simulink model "scdairframe"  (Simulink 6.0)
settings: Solver=ode45  SolverMode=SingleTasking  StartTime=0.0  StopTime=10.0  RelTol=1e-3  AbsTol=1e-6
PreLoadFcn:
  | aero_guid_dat
undefined symbols (not defined in the file or in its folder): Cm_alpha, Cm_el, Cm_q, Cx_alpha, Cz_alpha, Cz_el, d_ref, g, h_ini, S_ref, Thrust, x_ini
libraries: aerospace x3
settings Model: Creator=The Mathworks Inc.  LastModifiedBy=jglass  ExtModeTrigMode=oneshot  ExtModeArmWhenConnect=off  ExtModeAutoUpdateStatusClock=off
settings DataIOCC: LimitDataPoints=off  SignalLoggingName=sigsOut
settings OptimizationCC: BlockReduction=off  BooleanDataType=off
settings DebuggingCC: CheckExecutionContextPreStartOutputMsg=on  CheckExecutionContextRuntimeOutputMsg=on  SolverPrmCheckMsg=none
settings HardwareCC: TargetUnknown=on
settings SFSimCC: SFSimApplyToAllLibs=on  SFSimBuildMode=Incremental

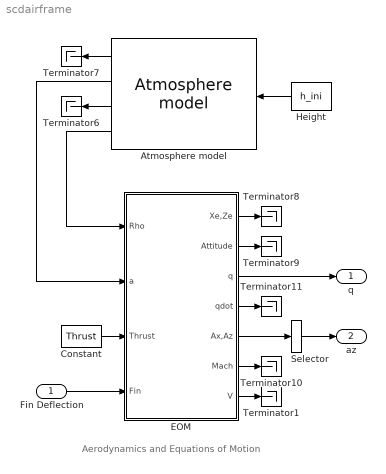
== system scdairframe ==
  note: Aerodynamics and Equations of Motion
  Fin Deflection : Inport  LatchInput=off
  Atmosphere model : aerospace/Atmosphere/Atmosphere model  Orientation=left
  Constant : Constant  Value=Thrust
  EOM : Subsystem  PropExecContextAcrossSSBoundary=on
  Height : Constant  Orientation=left  Value=h_ini
  Selector : Selector  Elements=[2]  InputPortWidth=2
  Terminator{1,6..11} (7 alike) : Terminator
  q : Outport  InitialOutput=0
  az : Outport  Port=2  InitialOutput=0
  wires:
  Height/1 -> Atmosphere model/1
  Atmosphere model/1 -> Terminator7/1
  Atmosphere model/3 -> Terminator6/1
  Constant/1 -> EOM/3(Thrust)
  Fin Deflection/1 -> EOM/4(Fin)
  EOM/1(Xe,Ze) -> Terminator8/1
  EOM/2(Attitude) -> Terminator9/1
  EOM/3(q) -> q/1
  EOM/4(qdot) -> Terminator11/1
  EOM/5(Ax,Az) -> Selector/1
  EOM/6(Mach) -> Terminator10/1
  Atmosphere model/4 -> EOM/1(Rho)
  Atmosphere model/2 -> EOM/2(a)
  Selector/1 -> az/1
  EOM/7(V) -> Terminator1/1

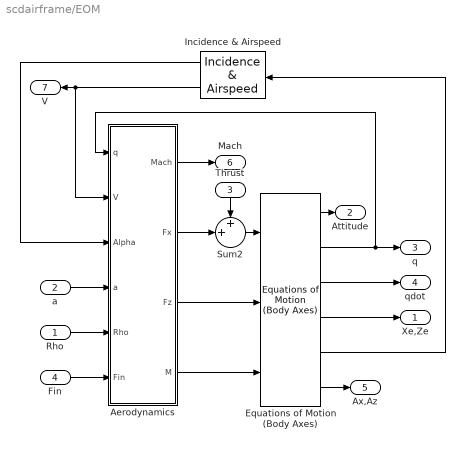
== system scdairframe/EOM ==
  Rho : Inport  LatchInput=off
  a : Inport  Port=2  LatchInput=off
  Thrust : Inport  Orientation=down  Port=3  LatchInput=off
  Fin : Inport  Port=4  LatchInput=off
  " Equations of Motion (Body Axes)" : aerospace/3DoF Equations of Motion / Equations of Motion (Body Axes)  v_ini=v_ini  theta_ini=theta_ini  alpha_ini=alpha_ini  q_ini=q_ini  pos_ini=[x_ini -h_ini]  mass=mass  Iyy=Iyy  g=g
  Aerodynamics : Subsystem  PropExecContextAcrossSSBoundary=on
  Incidence & Airspeed : aerospace/3DoF Equations of Motion /Incidence  & Airspeed  Orientation=left
  Sum2 : Sum  Inputs=++|  SaturateOnIntegerOverflow=on  InputSameDT=on
  Xe,Ze : Outport  InitialOutput=0
  Attitude : Outport  Port=2  InitialOutput=0
  q : Outport  Port=3  InitialOutput=0
  qdot : Outport  Port=4  InitialOutput=0
  Ax,Az : Outport  Port=5  InitialOutput=0
  Mach : Outport  Port=6  InitialOutput=0
  V : Outport  Orientation=left  Port=7  InitialOutput=0
  wires:
  " Equations of Motion (Body Axes)"/5 -> Incidence & Airspeed/1
  " Equations of Motion (Body Axes)"/6 -> Ax,Az/1
  " Equations of Motion (Body Axes)"/4 -> Xe,Ze/1
  " Equations of Motion (Body Axes)"/1 -> Attitude/1
  " Equations of Motion (Body Axes)"/3 -> qdot/1
  " Equations of Motion (Body Axes)"/2 -> Aerodynamics/1(q), q/1
  Thrust/1 -> Sum2/1
  Aerodynamics/2(Fx) -> Sum2/2
  Aerodynamics/3(Fz) -> " Equations of Motion (Body Axes)"/2
  Incidence & Airspeed/2 -> Aerodynamics/2(V), V/1
  Fin/1 -> Aerodynamics/6(Fin)
  a/1 -> Aerodynamics/4(a)
  Rho/1 -> Aerodynamics/5(Rho)
  Incidence & Airspeed/1 -> Aerodynamics/3(Alpha)
  Sum2/1 -> " Equations of Motion (Body Axes)"/1
  Aerodynamics/4(" M") -> " Equations of Motion (Body Axes)"/3
  Aerodynamics/1(" Mach") -> Mach/1

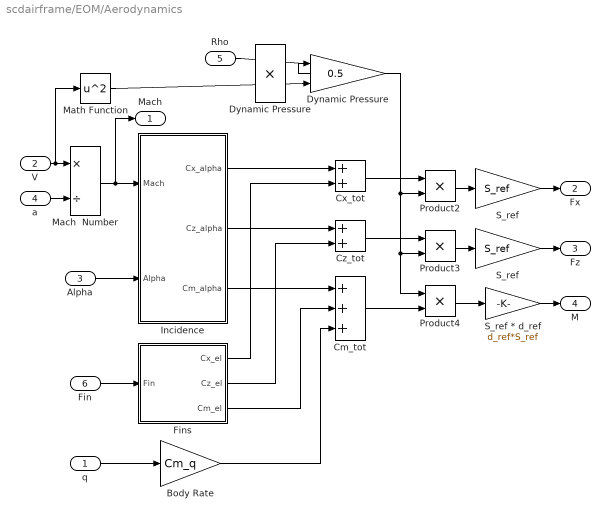
== system scdairframe/EOM/Aerodynamics ==
  q : Inport  LatchInput=off
  V : Inport  Port=2  LatchInput=off
  Alpha : Inport  Port=3  LatchInput=off
  a : Inport  Port=4  LatchInput=off
  Rho : Inport  Port=5  LatchInput=off
  Fin : Inport  Port=6  LatchInput=off
  Body Rate : Gain  Gain=Cm_q  SaturateOnIntegerOverflow=on
  Cm_tot : Sum  Inputs=+++  SaturateOnIntegerOverflow=on  InputSameDT=on
  Cx_tot : Sum  SaturateOnIntegerOverflow=on  InputSameDT=on
  Cz_tot : Sum  SaturateOnIntegerOverflow=on  InputSameDT=on
  Dynamic Pressure : Gain  Gain=0.5  SaturateOnIntegerOverflow=on
  Dynamic Pressure : Product  SaturateOnIntegerOverflow=on  InputSameDT=on
  Fins : Subsystem  PropExecContextAcrossSSBoundary=on
  Incidence : Subsystem  PropExecContextAcrossSSBoundary=on
  Mach  Number : Product  Inputs=*/  SaturateOnIntegerOverflow=on  InputSameDT=on
  Math Function : Math  Operator=square  SaturateOnIntegerOverflow=on
  Product2 : Product  SaturateOnIntegerOverflow=on  InputSameDT=on
  Product3 : Product  SaturateOnIntegerOverflow=on  InputSameDT=on
  Product4 : Product  SaturateOnIntegerOverflow=on  InputSameDT=on
  S_ref : Gain  Gain=S_ref  SaturateOnIntegerOverflow=on
  S_ref * d_ref : Gain  Gain=d_ref*S_ref  SaturateOnIntegerOverflow=on
  "S_ref " : Gain  Gain=S_ref  SaturateOnIntegerOverflow=on
  " Mach" : Outport  InitialOutput=0
  Fx : Outport  Port=2  InitialOutput=[0]
  Fz : Outport  Port=3  InitialOutput=0
  " M" : Outport  Port=4  InitialOutput=0
  wires:
  Mach  Number/1 -> Incidence/1(Mach), " Mach"/1
  q/1 -> Body Rate/1
  Cm_tot/1 -> Product4/2
  Product4/1 -> S_ref * d_ref/1
  S_ref * d_ref/1 -> " M"/1
  Fin/1 -> Fins/1(Fin)
  "S_ref "/1 -> Fz/1
  Product3/1 -> "S_ref "/1
  S_ref/1 -> Fx/1
  Product2/1 -> S_ref/1
  Cz_tot/1 -> Product3/1
  Cx_tot/1 -> Product2/1
  Alpha/1 -> Incidence/2(Alpha)
  a/1 -> Mach  Number/2
  Body Rate/1 -> Cm_tot/3
  Fins/3(Cm_el) -> Cm_tot/2
  Incidence/3(Cm_alpha) -> Cm_tot/1
  Fins/2(Cz_el) -> Cz_tot/2
  Incidence/2(Cz_alpha) -> Cz_tot/1
  Fins/1(Cx_el) -> Cx_tot/2
  Incidence/1(Cx_alpha) -> Cx_tot/1
  V/1 -> Mach  Number/1, Math Function/1
  Dynamic Pressure/1 -> Product4/1, Product3/2, Product2/2
  Dynamic Pressure/1 -> Dynamic Pressure/1
  Rho/1 -> Dynamic Pressure/1
  Math Function/1 -> Dynamic Pressure/2

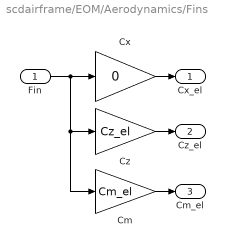
== system scdairframe/EOM/Aerodynamics/Fins ==
  Fin : Inport  LatchInput=off
  Cm : Gain  Gain=Cm_el  SaturateOnIntegerOverflow=on
  Cx : Gain  Gain=0  SaturateOnIntegerOverflow=on
  Cz : Gain  Gain=Cz_el  SaturateOnIntegerOverflow=on
  Cx_el : Outport  InitialOutput=0
  Cz_el : Outport  Port=2  InitialOutput=0
  Cm_el : Outport  Port=3  InitialOutput=0
  wires:
  Cz/1 -> Cz_el/1
  Cm/1 -> Cm_el/1
  Cx/1 -> Cx_el/1
  Fin/1 -> Cz/1, Cm/1, Cx/1

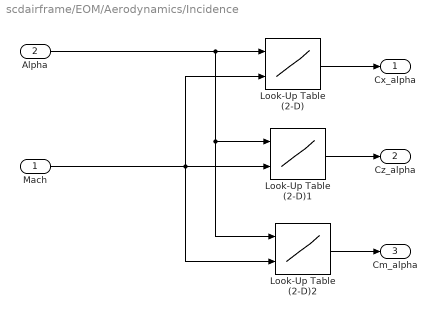
== system scdairframe/EOM/Aerodynamics/Incidence ==
  Mach : Inport  LatchInput=off
  Alpha : Inport  Port=2  LatchInput=off
  Look-Up Table (2-D) : Lookup2D  DialogController=Simulink.DDGSource  RowIndex=alpha_vec  ColumnIndex=Mach_vec  OutputValues=Cx_alpha  SaturateOnIntegerOverflow=on
  Look-Up Table (2-D)1 : Lookup2D  DialogController=Simulink.DDGSource  RowIndex=alpha_vec  ColumnIndex=Mach_vec  OutputValues=Cz_alpha  SaturateOnIntegerOverflow=on
  Look-Up Table (2-D)2 : Lookup2D  DialogController=Simulink.DDGSource  RowIndex=alpha_vec  ColumnIndex=Mach_vec  OutputValues=Cm_alpha  SaturateOnIntegerOverflow=on
  Cx_alpha : Outport  InitialOutput=0
  Cz_alpha : Outport  Port=2  InitialOutput=0
  Cm_alpha : Outport  Port=3  InitialOutput=0
  wires:
  Mach/1 -> Look-Up Table (2-D)2/2, Look-Up Table (2-D)1/2, Look-Up Table (2-D)/2
  Alpha/1 -> Look-Up Table (2-D)2/1, Look-Up Table (2-D)1/1, Look-Up Table (2-D)/1
  Look-Up Table (2-D)2/1 -> Cm_alpha/1
  Look-Up Table (2-D)1/1 -> Cz_alpha/1
  Look-Up Table (2-D)/1 -> Cx_alpha/1
